simulink model "AW_test"  (R2015a)
settings: Solver=ode5  StartTime=0.0  StopTime=0.5  FixedStep=1e-5  MaxStep=1e-4  RelTol=1e-3
values from neighbouring files (symbols this model uses):
  Af = [-15.9802071238 -2566.97948561 -96.8709621573 -60.7443875975 -54.1893771527 41.3534774927 -111.758131839 -5.18957577709 4.71062280365 61.452788526 0.0297969919136 0.177289731224 ... (144 elements, 12x12)]    [identified_t1_full.mat]
  Ak = [-672.634870495 -2626.58972998 -46.1193303275 25.5793500122 108.891317034 -102.718752792 -245.794654799 -577.315326704 39.8827087547 153.58157137 60.36854216 -207.81122515 ... (144 elements, 12x12)]    [controller.mat]    (also in main_matlab_single_step.m = rlqg.A)
  Bf = [-0.242989780525 -0.0299322746251 0.321554597542 0.228133316924 0.286172349315 -0.305996080434 -0.00624937622709 0.299905571178 0.0491887335661 0.146540635678 -0.0583489322764 0.229737532171 ... (24 elements, 12x2)]    [identified_t1_full.mat]
  Bk = [0.204306341627 1.11161335273 -0.324978673641 2.85402340631 -4.5813117605 2.97328839236 -0.174709893359 1.31662160979 2.94898293865 13.5567055967 -0.791381118401 0.0552385579013]    [controller.mat]    (also in main_matlab_single_step.m = rlqg.B)
  Cf = [11.6526185223 -2.27862995386 -17.2646212697 -3.07480298339 -1.84306279106 6.13326135217 -7.61687548654 -1.01458329844 1.12240644674 6.24617551809 15.4271955414 -17.0295297306]    [identified_t1_full.mat]
  Ck = [534.788956442 909.016401092 107.069958755 -410.092366717 -1097.26369634 478.53061829 -894.210554118 460.341899649 -450.064931583 371.993181033 532.787728171 55.8162878584 ... (24 elements, 2x12)]    [controller.mat]    (also in main_matlab_single_step.m = rlqg.C)
  Dk = [0 0]    [controller.mat]    (also in main_matlab_single_step.m = rlqg.D)
  GAMA1 = [-194.408609479 -2487.50601065 -57.1875850511 32.5640067864 -7.63693657744 -32.2406611442 -51.9156271093 -28.5024197504 20.1323492864 223.767501184 6.61156787132 -179.387575011 ... (576 elements, 24x24)]    [GAMA.mat]    (also in main_matlab_single_step.m = value(GAMA1); matlab.mat = [-204.738588884 -2421.75667304 -56.7590828092 132.094687962 ; matlab1.mat = [-82.2603255445 -2453.28100145 -97.6763768026 30.4858712578 )
  GAMA2 = [679.145432754 35.4785406858 -453.952353099 -329.010306868 -420.143585457 407.611641944 74.4677139316 88.8473791446 -231.86740129 -192.650053044 226.054657231 -495.830491749 ... (48 elements, 24x2)]    [GAMA.mat]    (also in main_matlab_single_step.m = value(GAMA2); matlab.mat = [-0.304779347057 -0.0633962985914 0.174246483556 0.110183261; matlab1.mat = [-0.0846006774632 -0.183440762718 0.0792576002981 0.00450245)
  GAMA3 = [8.87625764129 0.123008382436 -0.0879151562066 -2.72880349441 4.45690329049 -3.58069668026 3.05184819083 -1.61967389164 -3.23580060446 -12.2546008369 2.46260777544 -0.443190324065 ... (336 elements, 14x24)]    [GAMA.mat]    (also in main_matlab_single_step.m = value(GAMA3); matlab.mat = [24.3561205415 -9.43097581907 -0.378907903598 -1.18975703693; matlab1.mat = [10.6364854899 -4.70664386399 0.177456161363 -1.13126094774 )
  GAMA4 = [0 0 0 0 0 0 0 0 0 0 0 0 ... (28 elements, 14x2)]    [GAMA.mat]    (also in main_matlab_single_step.m = value(GAMA4); matlab.mat = [-0.00551391599343 -0.00506940014205 0.00017568156106 -0.000; matlab1.mat = [-0.0106677802601 0.000420174623854 0.00161102848178 -0.0039)
  Hf = [-0.00603819148621 -0.0121645329261 0.00178372873077 -0.020497816306 0.0668191856228 0.0461443111066 0.00197372154204 -0.00747704137343 -0.135635344699 -0.102773865384 0.0647006981549 0.0468916096625]    [identified_t1_full.mat]
  nc = dum5(1,2)    [main_matlab_single_step.m]
  nu = 2    [main_matlab_single_step.m]
settings Model: Creator=p4wp4w  LastModifiedBy=Ablah

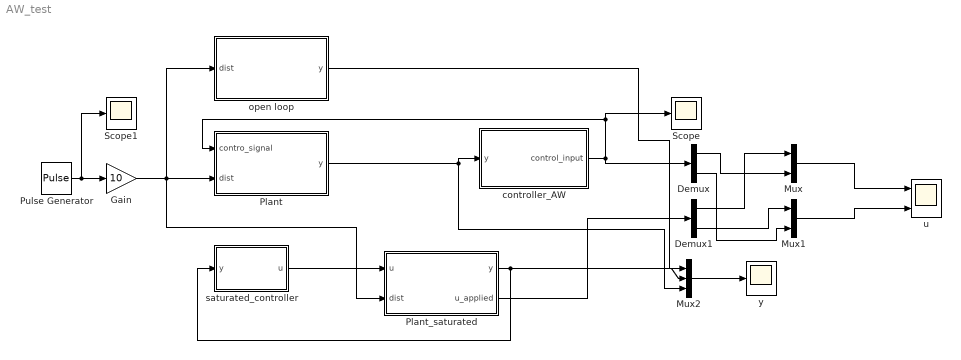
== system AW_test ==
  Demux : Demux  Outputs=2
  Demux1 : Demux  Outputs=2
  Gain : Gain  Gain=10
  Mux : Mux  Inputs=2
  Mux1 : Mux  Inputs=2
  Mux2 : Mux  Inputs=3
  Plant : Subsystem
  Plant_saturated : Subsystem
  Pulse Generator : DiscretePulseGenerator  PulseType=Time based  Period=0.5  PulseWidth=10
  Scope : Scope
      settings: SaveName=ScopeData4
  Scope1 : Scope
      settings: SaveName=ScopeData5
  controller_AW : Subsystem
  open loop : Subsystem
  "saturated_controller " : Subsystem
  u : Scope  NumInputPorts=2
      settings: ShowLegends=on  YMin=-0.45~-0.2  YMax=0.2~0.125
  y : Scope
      settings: YMin=-0.03  YMax=0.03
  wires:
  Plant/1(y) -> controller_AW/1(y), Mux2/3
  controller_AW/1("control_input ") -> Scope/1, Plant/1(contro_signal), Demux/1
  Pulse Generator/1 -> Scope1/1, Gain/1
  "saturated_controller "/1(u) -> Plant_saturated/1(u)
  Plant_saturated/1(y) -> Mux2/2, "saturated_controller "/1(y)
  Demux1/1 -> Mux/1
  Demux/1 -> Mux/2
  Demux1/2 -> Mux1/1
  Demux/2 -> Mux1/2
  Mux/1 -> u/1
  Mux1/1 -> u/2
  Plant_saturated/2(u_applied) -> Demux1/1
  Gain/1 -> Plant_saturated/2(dist), open loop/1(dist), Plant/2(dist)
  Mux2/1 -> y/1
  open loop/1(y) -> Mux2/1

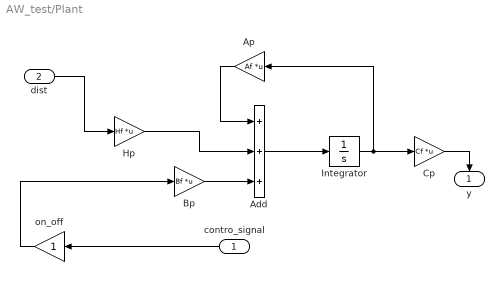
== system AW_test/Plant ==
  contro_signal : Inport
  dist : Inport  Port=2
  Add : Sum  Inputs=+++
  Ap : Gain  Gain=Af  Multiplication=Matrix(K*u)
  Bp : Gain  Gain=Bf  Multiplication=Matrix(K*u)
  Cp : Gain  Gain=Cf  Multiplication=Matrix(K*u)
  Hp : Gain  Gain=Hf  Multiplication=Matrix(K*u)
  Integrator : Integrator
  on_off : Gain
  y : Outport
  wires:
  Add/1 -> Integrator/1
  Cp/1 -> y/1
  Hp/1 -> Add/2
  on_off/1 -> Bp/1
  Integrator/1 -> Cp/1, Ap/1
  Ap/1 -> Add/1
  Bp/1 -> Add/3
  dist/1 -> Hp/1
  contro_signal/1 -> on_off/1

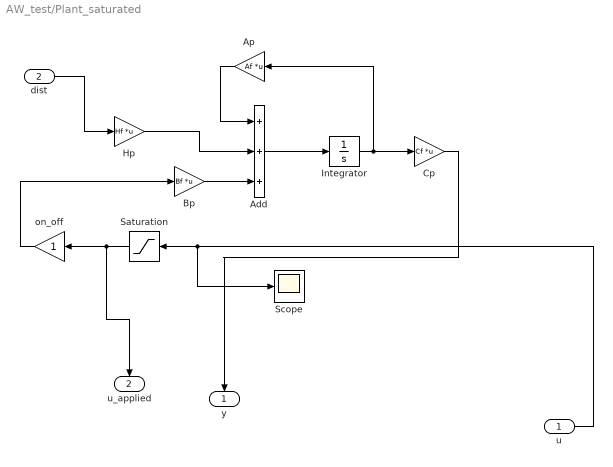
== system AW_test/Plant_saturated ==
  u : Inport
  dist : Inport  Port=2
  Add : Sum  Inputs=+++
  Ap : Gain  Gain=Af  Multiplication=Matrix(K*u)
  Bp : Gain  Gain=Bf  Multiplication=Matrix(K*u)
  Cp : Gain  Gain=Cf  Multiplication=Matrix(K*u)
  Hp : Gain  Gain=Hf  Multiplication=Matrix(K*u)
  Integrator : Integrator
  Saturation : Saturate  UpperLimit=2  LowerLimit=-2
  Scope : Scope
      settings: YMin=-10  YMax=10  SaveName=ScopeData2
  on_off : Gain
  y : Outport
  u_applied : Outport  Port=2
  wires:
  dist/1 -> Hp/1
  Bp/1 -> Add/3
  u/1 -> Scope/1, Saturation/1
  Ap/1 -> Add/1
  Saturation/1 -> u_applied/1, on_off/1
  Integrator/1 -> Ap/1, Cp/1
  on_off/1 -> Bp/1
  Hp/1 -> Add/2
  Cp/1 -> y/1
  Add/1 -> Integrator/1

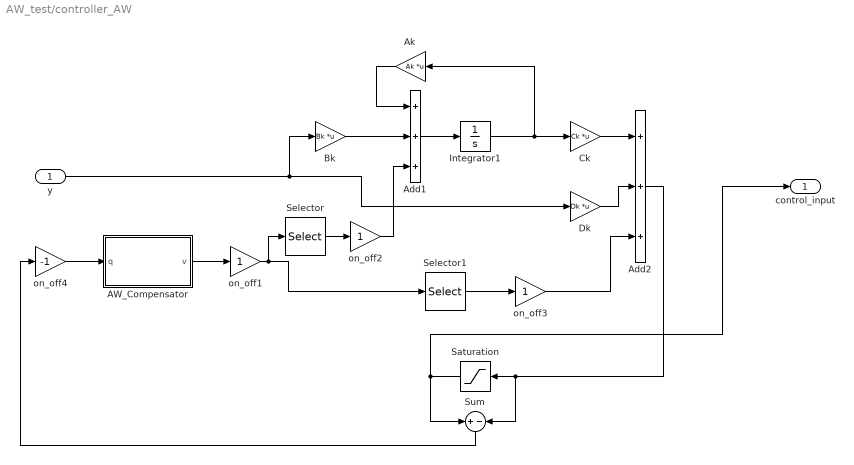
== system AW_test/controller_AW ==
  y : Inport
  AW_Compensator : Subsystem
  Add1 : Sum  Inputs=+++
  Add2 : Sum  Inputs=+++
  Ak : Gain  Gain=Ak  Multiplication=Matrix(K*u)
  Bk : Gain  Gain=Bk  Multiplication=Matrix(K*u)
  Ck : Gain  Gain=Ck  Multiplication=Matrix(K*u)
  Dk : Gain  Gain=Dk  Multiplication=Matrix(K*u)
  Integrator1 : Integrator
  Saturation : Saturate  UpperLimit=2  LowerLimit=-2
  Selector : Selector  InputPortWidth=nc+nu  Indices=[1:nc]
  Selector1 : Selector  InputPortWidth=nc+nu  Indices=[nc+1:nc+nu]
  Sum : Sum  Inputs=+|-
  on_off1 : Gain
  on_off2 : Gain
  on_off3 : Gain
  on_off4 : Gain  Gain=-1
  "control_input " : Outport
  wires:
  Ck/1 -> Add2/1
  Add1/1 -> Integrator1/1
  Ak/1 -> Add1/1
  AW_Compensator/1(v) -> on_off1/1
  Bk/1 -> Add1/2
  Integrator1/1 -> Ck/1, Ak/1
  Dk/1 -> Add2/2
  y/1 -> Dk/1, Bk/1
  Sum/1 -> on_off4/1
  on_off2/1 -> Add1/3
  on_off3/1 -> Add2/3
  Selector1/1 -> on_off3/1
  on_off1/1 -> Selector/1, Selector1/1
  Selector/1 -> on_off2/1
  on_off4/1 -> AW_Compensator/1(q)
  Saturation/1 -> "control_input "/1, Sum/1
  Add2/1 -> Sum/2, Saturation/1

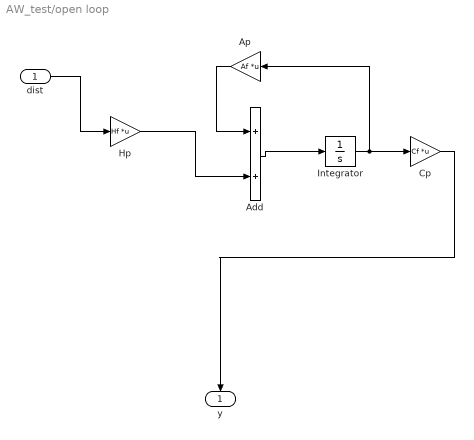
== system AW_test/open loop ==
  dist : Inport
  Add : Sum
  Ap : Gain  Gain=Af  Multiplication=Matrix(K*u)
  Cp : Gain  Gain=Cf  Multiplication=Matrix(K*u)
  Hp : Gain  Gain=Hf  Multiplication=Matrix(K*u)
  Integrator : Integrator
  y : Outport
  wires:
  dist/1 -> Hp/1
  Ap/1 -> Add/1
  Integrator/1 -> Ap/1, Cp/1
  Hp/1 -> Add/2
  Cp/1 -> y/1
  Add/1 -> Integrator/1

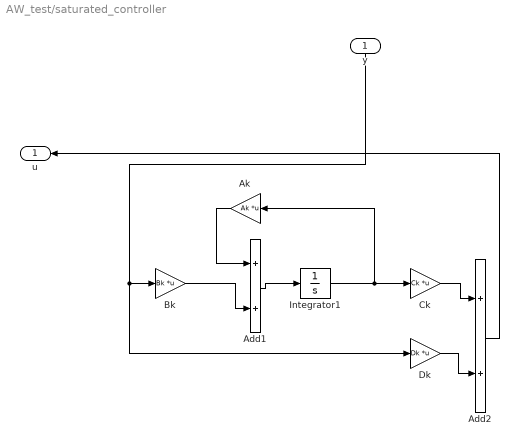
== system AW_test/saturated_controller  ==
  y : Inport
  Add1 : Sum
  Add2 : Sum
  Ak : Gain  Gain=Ak  Multiplication=Matrix(K*u)
  Bk : Gain  Gain=Bk  Multiplication=Matrix(K*u)
  Ck : Gain  Gain=Ck  Multiplication=Matrix(K*u)
  Dk : Gain  Gain=Dk  Multiplication=Matrix(K*u)
  Integrator1 : Integrator
  u : Outport
  wires:
  Bk/1 -> Add1/2
  Add1/1 -> Integrator1/1
  Ck/1 -> Add2/1
  Dk/1 -> Add2/2
  Integrator1/1 -> Ck/1, Ak/1
  Add2/1 -> u/1
  Ak/1 -> Add1/1
  y/1 -> Bk/1, Dk/1

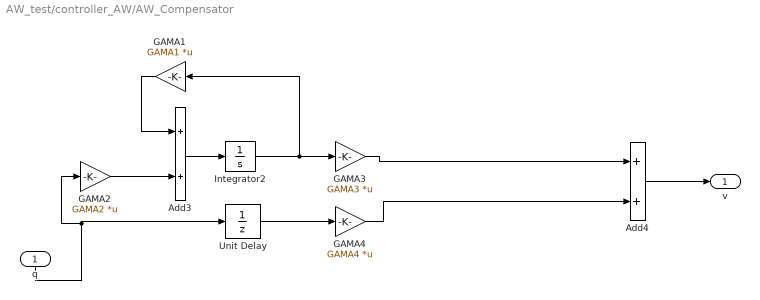
== system AW_test/controller_AW/AW_Compensator ==
  q : Inport
  Add3 : Sum
  Add4 : Sum
  GAMA1 : Gain  Gain=GAMA1  Multiplication=Matrix(K*u)
  GAMA2 : Gain  Gain=GAMA2  Multiplication=Matrix(K*u)
  GAMA3 : Gain  Gain=GAMA3  Multiplication=Matrix(K*u)
  GAMA4 : Gain  Gain=GAMA4  Multiplication=Matrix(K*u)
  Integrator2 : Integrator
  Unit Delay : UnitDelay  SampleTime=-1
  v : Outport
  wires:
  Add3/1 -> Integrator2/1
  GAMA3/1 -> Add4/1
  GAMA1/1 -> Add3/1
  Integrator2/1 -> GAMA1/1, GAMA3/1
  GAMA2/1 -> Add3/2
  GAMA4/1 -> Add4/2
  Add4/1 -> v/1
  q/1 -> Unit Delay/1, GAMA2/1
  Unit Delay/1 -> GAMA4/1
